simulink model "motor_kit_sim_20MHz"  (R2021b)
settings: Solver=VariableStepAuto  StartTime=0.0  StopTime=10*62.5E-6  RelTol=1e-3  EnableMultiTasking=on
PreLoadFcn:
  | setup_motor_kit_sim_20MHz;
InitFcn:
  | setup_motor_kit_sim_20MHz;
values from neighbouring files (symbols this model uses):
  DSPBASampleTime = 0.05e-6    (= 5e-08)    [setup_motor_kit_sim_20MHz.m]
  wordLength = 16    [setup_motor_kit_sim_20MHz.m]
undefined symbols (not defined in the file or in its folder): AdvDSPBChannelOutDisplay, dpoly, dspba_ChannelInVis, dspba_ChannelOutVis, dspba_internal_get_channel_ports, evalAionMaskParam, latency, primtype, value, x
libraries: DSPBAPrim x324, DSPBAModelBus x25, DSPBABase x7, dspsrcs4 x3, simulink x3, DSPBAUtilities x1
(part 2 of 5)

== system motor_kit_sim_20MHz/MotorModel/Current_scale_64_2 ==
  note: Motor phase currents 16 bits Sigma-Delta ADC (ADC interface:16 bits . Interface rtl: ip\ssg_emb_sd_adc ) : 1024 counts/A. Data type:sfix16_En10. Convert this value to range 0 to 1 (ufix16_En16). 2^16/1024 = 64; 2^15/1024 = 32. This means -32A will be 0 and 32A will be 1.
      | Schematic page 12: +/-32A current measurement. Current is sensed across 0.01 resistor. I=V/R = V/0.01 = 100*V
      | Motor phase currents Intel MAX10 ADC: 81.9 counts/A, convert this value to 16 bits, same as Sigma-Delta ADC:
      | MAX10 ADC read back value * 1024/81.9 = MAX10 ADC read back value * 12803/1024
  Current_range_int16 : Inport
  Current_sfix16_En10 : Inport  Port=2
  Add1 : DSPBAPrim/Add  primtype=add  nInputs=evalAionMaskParam(gcb,'value',1)  nOutputs=1  omode=Inherit via internal rule with word growth  otype=sfix(16)  scale=2^-15  rndmethod=Unbiased  factor=1  satmethod=Symmetric  shift_vec=[0 1 2 -1]  value=2  inPortNames=[' '; ' ';]  outPortNames=[' ']  dspbaimage=dspba_prim.svg  text=fprintf('+');  style=Optimised  visibilities=1032+2^17+2^18+2^19  genFPC=off  floatRounding=correct  advOptions=[]  version=20211007
  Const1 : DSPBAPrim/Const  primtype=const  nInputs=0  nOutputs=1  omode=Specify via dialog  otype=DataType  scale=constScaleFraction  rndmethod=Unbiased  factor=1  satmethod=Symmetric  shift_vec=[0 1 2 -1]  value=1/2  inPortNames=['+'; '+';]  outPortNames=[' ']  dspbaimage=dspba_prim.svg  text=fprintf('%s', num2str(value));  style=Optimised  visibilities=8 + 1024  floatPrecision=float32_m23  warnSaturation=on  version=20211007  SampleTime=inf
  Convert4 : DSPBAPrim/Convert  primtype=convert  nInputs=1  nOutputs=1  omode=Specify via dialog  otype=DataTypeFraction  scale=constScaleFraction  rndmethod=Biased  factor=1  satmethod=None  shift_vec=[0 1 2 -1]  value=round([0:255]/17)  inPortNames=[' '; ' ';]  outPortNames=[' '; 'c']  dspbaimage=dspba_prim_wide.svg  text=fprintf('convert');  style=Optimised  visibilities=8+64+256+2^17  clipdetect=off  floatPrecision=float32_m23  advOptions=[]  version=20211007
  Divide : DSPBAPrim/Divide  primtype=divide  nInputs=2  nOutputs=1  omode=Inherit via internal rule  otype=sfix(16)  scale=2^-15  rndmethod=Unbiased  factor=1  satmethod=Symmetric  shift_vec=[0 1 2 -1]  value=round([0:255]/17)  inPortNames=[' '; ' ';]  outPortNames=[' ']  dspbaimage=dspba_prim.svg  text=fprintf('a\n----\nb');  style=Optimised  visibilities=8+2^17+2^18  floatRounding=correct  intDivider=off  advOptions=[]  version=20211007
  GPIn : DSPBAPrim/GPIn  primtype=gpin  nInputs=evalAionMaskParam(gcb,'value',1)  nOutputs=evalAionMaskParam(gcb,'value',1)  omode=Inherit via internal rule  otype=sfix(16)  scale=2^-15  rndmethod=Unbiased  factor=1  satmethod=Symmetric  shift_vec=[0 1 2 -1]  value=1  inPortNames=[' ' ' ' ' ' ' ' ' ' ' ' ' ' ' ' ' ' ' ' ' ' ' ' ' ' ' ' ' ' ' ' ' ' ' ' ' ' ' ' ' ' ' ' ' ' ' ' ' ' ' ' ' ' ' ' ' ' ' ' ' ' ' ' ' ' ' ' ' ']'  outPortNames=[' ' ' ' ' ' ' ' ' ' ' ' ' ' ' ' ' ' ' ' ' ' ' ' ' ' ' ' ' ' ' ' ' ' ' ' ' ' ' ' ' ' ' ' ' ' ' ' ' ' ' ' ' ' ' ' ' ' ' ' ' ' ' ' ' ' ' ' ' ']'  dspbaimage=dspba_prim_channel_tall.svg  text=fprintf('GPIn');  style=Optimised  visibilities=1024  scheduleOrigin=off  version=20211214
  GPIn1 : DSPBAPrim/GPIn  primtype=gpin  nInputs=evalAionMaskParam(gcb,'value',1)  nOutputs=evalAionMaskParam(gcb,'value',1)  omode=Inherit via internal rule  otype=sfix(16)  scale=2^-15  rndmethod=Unbiased  factor=1  satmethod=Symmetric  shift_vec=[0 1 2 -1]  value=1  inPortNames=[' ' ' ' ' ' ' ' ' ' ' ' ' ' ' ' ' ' ' ' ' ' ' ' ' ' ' ' ' ' ' ' ' ' ' ' ' ' ' ' ' ' ' ' ' ' ' ' ' ' ' ' ' ' ' ' ' ' ' ' ' ' ' ' ' ' ' ' ' ']'  outPortNames=[' ' ' ' ' ' ' ' ' ' ' ' ' ' ' ' ' ' ' ' ' ' ' ' ' ' ' ' ' ' ' ' ' ' ' ' ' ' ' ' ' ' ' ' ' ' ' ' ' ' ' ' ' ' ' ' ' ' ' ' ' ' ' ' ' ' ' ' ' ']'  dspbaimage=dspba_prim_channel_tall.svg  text=fprintf('GPIn');  style=Optimised  visibilities=1024  scheduleOrigin=off  version=20211214
  GPOut : DSPBAPrim/GPOut  primtype=gpout  nInputs=evalAionMaskParam(gcb,'value',1)  nOutputs=evalAionMaskParam(gcb,'value',1)  omode=Inherit via internal rule  otype=sfix(16)  scale=2^-15  rndmethod=Unbiased  factor=1  satmethod=Symmetric  shift_vec=[0 1 2 -1]  value=1  inPortNames=[' ' ' ' ' ' ' ' ' ' ' ' ' ' ' ' ' ' ' ' ' ' ' ' ' ' ' ' ' ' ' ' ' ' ' ' ' ' ' ' ' ' ' ' ' ' ' ' ' ' ' ' ' ' ' ' ' ' ' ' ' ' ' ' ' ' ' ' ' ']'  outPortNames=[' ' ' ' ' ' ' ' ' ' ' ' ' ' ' ' ' ' ' ' ' ' ' ' ' ' ' ' ' ' ' ' ' ' ' ' ' ' ' ' ' ' ' ' ' ' ' ' ' ' ' ' ' ' ' ' ' ' ' ' ' ' ' ' ' ' ' ' ' ']'  dspbaimage=dspba_prim_channel_tall.svg  text=fprintf('GPOut');  style=Optimised  visibilities=1024  latency=13  version=20211214
  Mult : DSPBAPrim/Mult  primtype=mult  nInputs=2  nOutputs=1  omode=Inherit via internal rule  otype=sfix(16)  scale=2^-15  rndmethod=Unbiased  factor=1  satmethod=Symmetric  shift_vec=[0 1 2 -1]  value=0  inPortNames=[' '; ' ';]  outPortNames=[' ']  dspbaimage=dspba_prim.svg  text=fprintf('X');  style=Optimised  visibilities=8+2^18+2^19  floatPrecision=float32_m23  floatRounding=correct  advOptions=[]  version=20211007
  SynthesisInfo1 : DSPBAPrim/SynthesisInfo  primtype=synthinfo  nInputs=0  nOutputs=0  omode=Inherit via internal rule  otype=sfix(16)  scale=2^-15  rndmethod=Truncate  factor=1  satmethod=Symmetric  shift_vec=[0 1 2 -1]  value=99  inPortNames=[' '; ' ';]  outPortNames=[' ']  dspbaimage=dspba_prim_ctrl.jpg  text=fprintf('Style=%s', style);  style=Scheduled  visibilities=2^17+2^18+2^19+2^20  constraintPair=None  constraintRelation=>  constraintLimit=2  modelRefSign=+  modelRef=''  showSchedule=off  simulationMode=Use Global Value  resetMinimization=Conditional - On for ChannelIn/Out only  version=20220106
  "Fraction_ND_ufix16_En16 " : Outport
  wires:
  Mult/1 -> Convert4/1
  GPIn1/1 -> Add1/2
  Divide/1 -> Mult/1
  Current_range_int16/1 -> GPIn/1
  Add1/1 -> Mult/2
  Convert4/1 -> GPOut/1
  GPOut/1 -> "Fraction_ND_ufix16_En16 "/1
  GPIn/1 -> Divide/2, Add1/1
  Const1/1 -> Divide/1
  Current_sfix16_En10/1 -> GPIn1/1

== system motor_kit_sim_20MHz/MotorModel/Fraction_to_Pulse ==
  note: Subtract threshold once it is reached
  Fraction_ND_ufix16_En16 : Inport
  Add : DSPBAPrim/Add  primtype=add  nInputs=evalAionMaskParam(gcb,'value',1)  nOutputs=1  omode=Inherit via internal rule with word growth  otype=sfix(16)  scale=2^-15  rndmethod=Unbiased  factor=1  satmethod=Symmetric  shift_vec=[0 1 2 -1]  value=2  inPortNames=[' '; ' ';]  outPortNames=[' ']  dspbaimage=dspba_prim.svg  text=fprintf('+');  style=Optimised  visibilities=1032+2^17+2^18+2^19  genFPC=off  floatRounding=correct  advOptions=[]  version=20211007
  CmpGE : DSPBAPrim/CmpGE  primtype=cmpgte  nInputs=2  nOutputs=1  omode=boolean  otype=sfix(16)  scale=2^-15  rndmethod=Unbiased  factor=1  satmethod=Symmetric  shift_vec=[0 1 2 -1]  value=0  inPortNames=['a'; 'b';]  outPortNames=[' ']  dspbaimage=dspba_prim.svg  text=fprintf('a>=b');  style=Optimised  visibilities=0  advOptions=[]  version=20211007
  Const1 : DSPBAPrim/Const  primtype=const  nInputs=0  nOutputs=1  omode=Specify via dialog  otype=DataTypeFraction  scale=constScaleFraction  rndmethod=Unbiased  factor=1  satmethod=Symmetric  shift_vec=[0 1 2 -1]  value=1  inPortNames=['+'; '+';]  outPortNames=[' ']  dspbaimage=dspba_prim.svg  text=fprintf('%s', num2str(value));  style=Optimised  visibilities=8 + 1024  floatPrecision=float32_m23  warnSaturation=on  version=20211007  SampleTime=inf
  Const2 : DSPBAPrim/Const  primtype=const  nInputs=0  nOutputs=1  omode=Specify via dialog  otype=DataTypeFraction  scale=constScaleFraction  rndmethod=Unbiased  factor=1  satmethod=Symmetric  shift_vec=[0 1 2 -1]  value=0  inPortNames=['+'; '+';]  outPortNames=[' ']  dspbaimage=dspba_prim.svg  text=fprintf('%s', num2str(value));  style=Optimised  visibilities=8 + 1024  floatPrecision=float32_m23  warnSaturation=on  version=20211007  SampleTime=inf
  Const3 : DSPBAPrim/Const  primtype=const  nInputs=0  nOutputs=1  omode=Specify via dialog  otype=DataTypeFraction  scale=constScaleFraction  rndmethod=Unbiased  factor=1  satmethod=Symmetric  shift_vec=[0 1 2 -1]  value=1  inPortNames=['+'; '+';]  outPortNames=[' ']  dspbaimage=dspba_prim.svg  text=fprintf('%s', num2str(value));  style=Optimised  visibilities=8 + 1024  floatPrecision=float32_m23  warnSaturation=on  version=20211007  SampleTime=inf
  Convert4 : DSPBAPrim/Convert  primtype=convert  nInputs=1  nOutputs=1  omode=Specify via dialog  otype=sfix(18)  scale=constScaleFraction  rndmethod=Biased  factor=1  satmethod=None  shift_vec=[0 1 2 -1]  value=round([0:255]/17)  inPortNames=[' '; ' ';]  outPortNames=[' '; 'c']  dspbaimage=dspba_prim_wide.svg  text=fprintf('convert');  style=Optimised  visibilities=8+64+256+2^17  clipdetect=off  floatPrecision=float32_m23  advOptions=[]  version=20211007
  GPIn : DSPBAPrim/GPIn  primtype=gpin  nInputs=evalAionMaskParam(gcb,'value',1)  nOutputs=evalAionMaskParam(gcb,'value',1)  omode=Inherit via internal rule  otype=sfix(16)  scale=2^-15  rndmethod=Unbiased  factor=1  satmethod=Symmetric  shift_vec=[0 1 2 -1]  value=1  inPortNames=[' ' ' ' ' ' ' ' ' ' ' ' ' ' ' ' ' ' ' ' ' ' ' ' ' ' ' ' ' ' ' ' ' ' ' ' ' ' ' ' ' ' ' ' ' ' ' ' ' ' ' ' ' ' ' ' ' ' ' ' ' ' ' ' ' ' ' ' ' ']'  outPortNames=[' ' ' ' ' ' ' ' ' ' ' ' ' ' ' ' ' ' ' ' ' ' ' ' ' ' ' ' ' ' ' ' ' ' ' ' ' ' ' ' ' ' ' ' ' ' ' ' ' ' ' ' ' ' ' ' ' ' ' ' ' ' ' ' ' ' ' ' ' ']'  dspbaimage=dspba_prim_channel_tall.svg  text=fprintf('GPIn');  style=Optimised  visibilities=1024  scheduleOrigin=off  version=20211214
  GPOut : DSPBAPrim/GPOut  primtype=gpout  nInputs=evalAionMaskParam(gcb,'value',1)  nOutputs=evalAionMaskParam(gcb,'value',1)  omode=Inherit via internal rule  otype=sfix(16)  scale=2^-15  rndmethod=Unbiased  factor=1  satmethod=Symmetric  shift_vec=[0 1 2 -1]  value=1  inPortNames=[' ' ' ' ' ' ' ' ' ' ' ' ' ' ' ' ' ' ' ' ' ' ' ' ' ' ' ' ' ' ' ' ' ' ' ' ' ' ' ' ' ' ' ' ' ' ' ' ' ' ' ' ' ' ' ' ' ' ' ' ' ' ' ' ' ' ' ' ' ']'  outPortNames=[' ' ' ' ' ' ' ' ' ' ' ' ' ' ' ' ' ' ' ' ' ' ' ' ' ' ' ' ' ' ' ' ' ' ' ' ' ' ' ' ' ' ' ' ' ' ' ' ' ' ' ' ' ' ' ' ' ' ' ' ' ' ' ' ' ' ' ' ' ']'  dspbaimage=dspba_prim_channel_tall.svg  text=fprintf('GPOut');  style=Optimised  visibilities=1024  latency=0  version=20211214
  Mux : DSPBAPrim/Mux  primtype=mux  nInputs=evalAionMaskParam(gcb,'value',1)+1  nOutputs=1  omode=Inherit via internal rule  otype=sfix(16)  scale=2^-15  rndmethod=Unbiased  factor=1  satmethod=Symmetric  shift_vec=[0 1 2 -1]  value=2  inPortNames=['s'; 'd0'; 'd1'; 'd2'; 'd3'; 'd4'; 'd5'; 'd6'; 'd7'; 'd8'; 'd9';]  outPortNames=[' ']  dspbaimage=dspba_prim_tall.svg  text=fprintf('%s', primtype);  style=Optimised  visibilities=1032  version=20211007
  SampleDelay : DSPBAPrim/SampleDelay  primtype=sampdelay  nInputs=1  nOutputs=1  omode=Inherit via internal rule  otype=sfix(16)  scale=2^-15  rndmethod=Unbiased  factor=1  satmethod=Symmetric  shift_vec=[0 1 2 -1]  floatPrecision=float32_m23  value=1  inPortNames=[' '; ' ';]  outPortNames=[' ']  dspbaimage=dspba_prim.svg  text=dpoly(1, eye(1,value+1), 'z')  style=Optimised  visibilities=8 + 1024 + 2^17 + 2^18  flexible=off  slackgroup=0  augmented=0  version=20211007  advOptions=[]
  Sub : DSPBAPrim/Sub  primtype=sub  nInputs=2  nOutputs=1  omode=Inherit via internal rule with word growth  otype=sfix(17)  scale=2^-15  rndmethod=Unbiased  factor=1  satmethod=Symmetric  shift_vec=[0 1 2 -1]  value=0  inPortNames=['+'; '-';]  outPortNames=[' ']  dspbaimage=dspba_prim.svg  text=fprintf('-');  style=Optimised  visibilities=8+2^17+2^18  floatRounding=correct  advOptions=[]  version=20211007
  SynthesisInfo1 : DSPBAPrim/SynthesisInfo  primtype=synthinfo  nInputs=0  nOutputs=0  omode=Inherit via internal rule  otype=sfix(16)  scale=2^-15  rndmethod=Truncate  factor=1  satmethod=Symmetric  shift_vec=[0 1 2 -1]  value=99  inPortNames=[' '; ' ';]  outPortNames=[' ']  dspbaimage=dspba_prim_ctrl.jpg  text=fprintf('Style=%s', style);  style=Scheduled  visibilities=2^17+2^18+2^19+2^20  constraintPair=None  constraintRelation=>  constraintLimit=2  modelRefSign=+  modelRef=''  showSchedule=off  simulationMode=Use Global Value  resetMinimization=Conditional - On for ChannelIn/Out only  version=20220106
  "PulseDensity_Bool " : Outport
  wires:
  Mux/1 -> Sub/2
  CmpGE/1 -> GPOut/1, Mux/1
  GPIn/1 -> Sub/1
  Const2/1 -> Mux/2
  Const1/1 -> Mux/3
  Sub/1 -> Add/1
  Fraction_ND_ufix16_En16/1 -> GPIn/1
  GPOut/1 -> "PulseDensity_Bool "/1
  Add/1 -> Convert4/1
  Const3/1 -> CmpGE/2
  SampleDelay/1 -> Add/2, CmpGE/1
  Convert4/1 -> SampleDelay/1

== system motor_kit_sim_20MHz/MotorModel/Fraction_to_Pulse1 ==
  note: Subtract threshold once it is reached
  Fraction_ND_ufix16_En16 : Inport
  Add : DSPBAPrim/Add  primtype=add  nInputs=evalAionMaskParam(gcb,'value',1)  nOutputs=1  omode=Inherit via internal rule with word growth  otype=sfix(16)  scale=2^-15  rndmethod=Unbiased  factor=1  satmethod=Symmetric  shift_vec=[0 1 2 -1]  value=2  inPortNames=[' '; ' ';]  outPortNames=[' ']  dspbaimage=dspba_prim.svg  text=fprintf('+');  style=Optimised  visibilities=1032+2^17+2^18+2^19  genFPC=off  floatRounding=correct  advOptions=[]  version=20211007
  CmpGE : DSPBAPrim/CmpGE  primtype=cmpgte  nInputs=2  nOutputs=1  omode=boolean  otype=sfix(16)  scale=2^-15  rndmethod=Unbiased  factor=1  satmethod=Symmetric  shift_vec=[0 1 2 -1]  value=0  inPortNames=['a'; 'b';]  outPortNames=[' ']  dspbaimage=dspba_prim.svg  text=fprintf('a>=b');  style=Optimised  visibilities=0  advOptions=[]  version=20211007
  Const1 : DSPBAPrim/Const  primtype=const  nInputs=0  nOutputs=1  omode=Specify via dialog  otype=DataTypeFraction  scale=constScaleFraction  rndmethod=Unbiased  factor=1  satmethod=Symmetric  shift_vec=[0 1 2 -1]  value=1  inPortNames=['+'; '+';]  outPortNames=[' ']  dspbaimage=dspba_prim.svg  text=fprintf('%s', num2str(value));  style=Optimised  visibilities=8 + 1024  floatPrecision=float32_m23  warnSaturation=on  version=20211007  SampleTime=inf
  Const2 : DSPBAPrim/Const  primtype=const  nInputs=0  nOutputs=1  omode=Specify via dialog  otype=DataTypeFraction  scale=constScaleFraction  rndmethod=Unbiased  factor=1  satmethod=Symmetric  shift_vec=[0 1 2 -1]  value=0  inPortNames=['+'; '+';]  outPortNames=[' ']  dspbaimage=dspba_prim.svg  text=fprintf('%s', num2str(value));  style=Optimised  visibilities=8 + 1024  floatPrecision=float32_m23  warnSaturation=on  version=20211007  SampleTime=inf
  Const3 : DSPBAPrim/Const  primtype=const  nInputs=0  nOutputs=1  omode=Specify via dialog  otype=DataTypeFraction  scale=constScaleFraction  rndmethod=Unbiased  factor=1  satmethod=Symmetric  shift_vec=[0 1 2 -1]  value=1  inPortNames=['+'; '+';]  outPortNames=[' ']  dspbaimage=dspba_prim.svg  text=fprintf('%s', num2str(value));  style=Optimised  visibilities=8 + 1024  floatPrecision=float32_m23  warnSaturation=on  version=20211007  SampleTime=inf
  Convert4 : DSPBAPrim/Convert  primtype=convert  nInputs=1  nOutputs=1  omode=Specify via dialog  otype=sfix(18)  scale=constScaleFraction  rndmethod=Biased  factor=1  satmethod=None  shift_vec=[0 1 2 -1]  value=round([0:255]/17)  inPortNames=[' '; ' ';]  outPortNames=[' '; 'c']  dspbaimage=dspba_prim_wide.svg  text=fprintf('convert');  style=Optimised  visibilities=8+64+256+2^17  clipdetect=off  floatPrecision=float32_m23  advOptions=[]  version=20211007
  GPIn : DSPBAPrim/GPIn  primtype=gpin  nInputs=evalAionMaskParam(gcb,'value',1)  nOutputs=evalAionMaskParam(gcb,'value',1)  omode=Inherit via internal rule  otype=sfix(16)  scale=2^-15  rndmethod=Unbiased  factor=1  satmethod=Symmetric  shift_vec=[0 1 2 -1]  value=1  inPortNames=[' ' ' ' ' ' ' ' ' ' ' ' ' ' ' ' ' ' ' ' ' ' ' ' ' ' ' ' ' ' ' ' ' ' ' ' ' ' ' ' ' ' ' ' ' ' ' ' ' ' ' ' ' ' ' ' ' ' ' ' ' ' ' ' ' ' ' ' ' ']'  outPortNames=[' ' ' ' ' ' ' ' ' ' ' ' ' ' ' ' ' ' ' ' ' ' ' ' ' ' ' ' ' ' ' ' ' ' ' ' ' ' ' ' ' ' ' ' ' ' ' ' ' ' ' ' ' ' ' ' ' ' ' ' ' ' ' ' ' ' ' ' ' ']'  dspbaimage=dspba_prim_channel_tall.svg  text=fprintf('GPIn');  style=Optimised  visibilities=1024  scheduleOrigin=off  version=20211214
  GPOut : DSPBAPrim/GPOut  primtype=gpout  nInputs=evalAionMaskParam(gcb,'value',1)  nOutputs=evalAionMaskParam(gcb,'value',1)  omode=Inherit via internal rule  otype=sfix(16)  scale=2^-15  rndmethod=Unbiased  factor=1  satmethod=Symmetric  shift_vec=[0 1 2 -1]  value=1  inPortNames=[' ' ' ' ' ' ' ' ' ' ' ' ' ' ' ' ' ' ' ' ' ' ' ' ' ' ' ' ' ' ' ' ' ' ' ' ' ' ' ' ' ' ' ' ' ' ' ' ' ' ' ' ' ' ' ' ' ' ' ' ' ' ' ' ' ' ' ' ' ']'  outPortNames=[' ' ' ' ' ' ' ' ' ' ' ' ' ' ' ' ' ' ' ' ' ' ' ' ' ' ' ' ' ' ' ' ' ' ' ' ' ' ' ' ' ' ' ' ' ' ' ' ' ' ' ' ' ' ' ' ' ' ' ' ' ' ' ' ' ' ' ' ' ']'  dspbaimage=dspba_prim_channel_tall.svg  text=fprintf('GPOut');  style=Optimised  visibilities=1024  latency=0  version=20211214
  Mux : DSPBAPrim/Mux  primtype=mux  nInputs=evalAionMaskParam(gcb,'value',1)+1  nOutputs=1  omode=Inherit via internal rule  otype=sfix(16)  scale=2^-15  rndmethod=Unbiased  factor=1  satmethod=Symmetric  shift_vec=[0 1 2 -1]  value=2  inPortNames=['s'; 'd0'; 'd1'; 'd2'; 'd3'; 'd4'; 'd5'; 'd6'; 'd7'; 'd8'; 'd9';]  outPortNames=[' ']  dspbaimage=dspba_prim_tall.svg  text=fprintf('%s', primtype);  style=Optimised  visibilities=1032  version=20211007
  SampleDelay : DSPBAPrim/SampleDelay  primtype=sampdelay  nInputs=1  nOutputs=1  omode=Inherit via internal rule  otype=sfix(16)  scale=2^-15  rndmethod=Unbiased  factor=1  satmethod=Symmetric  shift_vec=[0 1 2 -1]  floatPrecision=float32_m23  value=1  inPortNames=[' '; ' ';]  outPortNames=[' ']  dspbaimage=dspba_prim.svg  text=dpoly(1, eye(1,value+1), 'z')  style=Optimised  visibilities=8 + 1024 + 2^17 + 2^18  flexible=off  slackgroup=0  augmented=0  version=20211007  advOptions=[]
  Sub : DSPBAPrim/Sub  primtype=sub  nInputs=2  nOutputs=1  omode=Inherit via internal rule with word growth  otype=sfix(17)  scale=2^-15  rndmethod=Unbiased  factor=1  satmethod=Symmetric  shift_vec=[0 1 2 -1]  value=0  inPortNames=['+'; '-';]  outPortNames=[' ']  dspbaimage=dspba_prim.svg  text=fprintf('-');  style=Optimised  visibilities=8+2^17+2^18  floatRounding=correct  advOptions=[]  version=20211007
  SynthesisInfo1 : DSPBAPrim/SynthesisInfo  primtype=synthinfo  nInputs=0  nOutputs=0  omode=Inherit via internal rule  otype=sfix(16)  scale=2^-15  rndmethod=Truncate  factor=1  satmethod=Symmetric  shift_vec=[0 1 2 -1]  value=99  inPortNames=[' '; ' ';]  outPortNames=[' ']  dspbaimage=dspba_prim_ctrl.jpg  text=fprintf('Style=%s', style);  style=Scheduled  visibilities=2^17+2^18+2^19+2^20  constraintPair=None  constraintRelation=>  constraintLimit=2  modelRefSign=+  modelRef=''  showSchedule=off  simulationMode=Use Global Value  resetMinimization=Conditional - On for ChannelIn/Out only  version=20220106
  "PulseDensity_Bool " : Outport
  wires:
  Mux/1 -> Sub/2
  CmpGE/1 -> GPOut/1, Mux/1
  GPIn/1 -> Sub/1
  Const2/1 -> Mux/2
  Const1/1 -> Mux/3
  Sub/1 -> Add/1
  Fraction_ND_ufix16_En16/1 -> GPIn/1
  GPOut/1 -> "PulseDensity_Bool "/1
  Add/1 -> Convert4/1
  Const3/1 -> CmpGE/2
  SampleDelay/1 -> Add/2, CmpGE/1
  Convert4/1 -> SampleDelay/1

== system motor_kit_sim_20MHz/MotorModel/Fraction_to_Pulse2 ==
  note: Subtract threshold once it is reached
  Fraction_ND_ufix16_En16 : Inport
  Add : DSPBAPrim/Add  primtype=add  nInputs=evalAionMaskParam(gcb,'value',1)  nOutputs=1  omode=Inherit via internal rule with word growth  otype=sfix(16)  scale=2^-15  rndmethod=Unbiased  factor=1  satmethod=Symmetric  shift_vec=[0 1 2 -1]  value=2  inPortNames=[' '; ' ';]  outPortNames=[' ']  dspbaimage=dspba_prim.svg  text=fprintf('+');  style=Optimised  visibilities=1032+2^17+2^18+2^19  genFPC=off  floatRounding=correct  advOptions=[]  version=20211007
  CmpGE : DSPBAPrim/CmpGE  primtype=cmpgte  nInputs=2  nOutputs=1  omode=boolean  otype=sfix(16)  scale=2^-15  rndmethod=Unbiased  factor=1  satmethod=Symmetric  shift_vec=[0 1 2 -1]  value=0  inPortNames=['a'; 'b';]  outPortNames=[' ']  dspbaimage=dspba_prim.svg  text=fprintf('a>=b');  style=Optimised  visibilities=0  advOptions=[]  version=20211007
  Const1 : DSPBAPrim/Const  primtype=const  nInputs=0  nOutputs=1  omode=Specify via dialog  otype=DataTypeFraction  scale=constScaleFraction  rndmethod=Unbiased  factor=1  satmethod=Symmetric  shift_vec=[0 1 2 -1]  value=1  inPortNames=['+'; '+';]  outPortNames=[' ']  dspbaimage=dspba_prim.svg  text=fprintf('%s', num2str(value));  style=Optimised  visibilities=8 + 1024  floatPrecision=float32_m23  warnSaturation=on  version=20211007  SampleTime=inf
  Const2 : DSPBAPrim/Const  primtype=const  nInputs=0  nOutputs=1  omode=Specify via dialog  otype=DataTypeFraction  scale=constScaleFraction  rndmethod=Unbiased  factor=1  satmethod=Symmetric  shift_vec=[0 1 2 -1]  value=0  inPortNames=['+'; '+';]  outPortNames=[' ']  dspbaimage=dspba_prim.svg  text=fprintf('%s', num2str(value));  style=Optimised  visibilities=8 + 1024  floatPrecision=float32_m23  warnSaturation=on  version=20211007  SampleTime=inf
  Const3 : DSPBAPrim/Const  primtype=const  nInputs=0  nOutputs=1  omode=Specify via dialog  otype=DataTypeFraction  scale=constScaleFraction  rndmethod=Unbiased  factor=1  satmethod=Symmetric  shift_vec=[0 1 2 -1]  value=1  inPortNames=['+'; '+';]  outPortNames=[' ']  dspbaimage=dspba_prim.svg  text=fprintf('%s', num2str(value));  style=Optimised  visibilities=8 + 1024  floatPrecision=float32_m23  warnSaturation=on  version=20211007  SampleTime=inf
  Convert4 : DSPBAPrim/Convert  primtype=convert  nInputs=1  nOutputs=1  omode=Specify via dialog  otype=sfix(18)  scale=constScaleFraction  rndmethod=Biased  factor=1  satmethod=None  shift_vec=[0 1 2 -1]  value=round([0:255]/17)  inPortNames=[' '; ' ';]  outPortNames=[' '; 'c']  dspbaimage=dspba_prim_wide.svg  text=fprintf('convert');  style=Optimised  visibilities=8+64+256+2^17  clipdetect=off  floatPrecision=float32_m23  advOptions=[]  version=20211007
  GPIn : DSPBAPrim/GPIn  primtype=gpin  nInputs=evalAionMaskParam(gcb,'value',1)  nOutputs=evalAionMaskParam(gcb,'value',1)  omode=Inherit via internal rule  otype=sfix(16)  scale=2^-15  rndmethod=Unbiased  factor=1  satmethod=Symmetric  shift_vec=[0 1 2 -1]  value=1  inPortNames=[' ' ' ' ' ' ' ' ' ' ' ' ' ' ' ' ' ' ' ' ' ' ' ' ' ' ' ' ' ' ' ' ' ' ' ' ' ' ' ' ' ' ' ' ' ' ' ' ' ' ' ' ' ' ' ' ' ' ' ' ' ' ' ' ' ' ' ' ' ']'  outPortNames=[' ' ' ' ' ' ' ' ' ' ' ' ' ' ' ' ' ' ' ' ' ' ' ' ' ' ' ' ' ' ' ' ' ' ' ' ' ' ' ' ' ' ' ' ' ' ' ' ' ' ' ' ' ' ' ' ' ' ' ' ' ' ' ' ' ' ' ' ' ']'  dspbaimage=dspba_prim_channel_tall.svg  text=fprintf('GPIn');  style=Optimised  visibilities=1024  scheduleOrigin=off  version=20211214
  GPOut : DSPBAPrim/GPOut  primtype=gpout  nInputs=evalAionMaskParam(gcb,'value',1)  nOutputs=evalAionMaskParam(gcb,'value',1)  omode=Inherit via internal rule  otype=sfix(16)  scale=2^-15  rndmethod=Unbiased  factor=1  satmethod=Symmetric  shift_vec=[0 1 2 -1]  value=1  inPortNames=[' ' ' ' ' ' ' ' ' ' ' ' ' ' ' ' ' ' ' ' ' ' ' ' ' ' ' ' ' ' ' ' ' ' ' ' ' ' ' ' ' ' ' ' ' ' ' ' ' ' ' ' ' ' ' ' ' ' ' ' ' ' ' ' ' ' ' ' ' ']'  outPortNames=[' ' ' ' ' ' ' ' ' ' ' ' ' ' ' ' ' ' ' ' ' ' ' ' ' ' ' ' ' ' ' ' ' ' ' ' ' ' ' ' ' ' ' ' ' ' ' ' ' ' ' ' ' ' ' ' ' ' ' ' ' ' ' ' ' ' ' ' ' ']'  dspbaimage=dspba_prim_channel_tall.svg  text=fprintf('GPOut');  style=Optimised  visibilities=1024  latency=0  version=20211214
  Mux : DSPBAPrim/Mux  primtype=mux  nInputs=evalAionMaskParam(gcb,'value',1)+1  nOutputs=1  omode=Inherit via internal rule  otype=sfix(16)  scale=2^-15  rndmethod=Unbiased  factor=1  satmethod=Symmetric  shift_vec=[0 1 2 -1]  value=2  inPortNames=['s'; 'd0'; 'd1'; 'd2'; 'd3'; 'd4'; 'd5'; 'd6'; 'd7'; 'd8'; 'd9';]  outPortNames=[' ']  dspbaimage=dspba_prim_tall.svg  text=fprintf('%s', primtype);  style=Optimised  visibilities=1032  version=20211007
  SampleDelay : DSPBAPrim/SampleDelay  primtype=sampdelay  nInputs=1  nOutputs=1  omode=Inherit via internal rule  otype=sfix(16)  scale=2^-15  rndmethod=Unbiased  factor=1  satmethod=Symmetric  shift_vec=[0 1 2 -1]  floatPrecision=float32_m23  value=1  inPortNames=[' '; ' ';]  outPortNames=[' ']  dspbaimage=dspba_prim.svg  text=dpoly(1, eye(1,value+1), 'z')  style=Optimised  visibilities=8 + 1024 + 2^17 + 2^18  flexible=off  slackgroup=0  augmented=0  version=20211007  advOptions=[]
  Sub : DSPBAPrim/Sub  primtype=sub  nInputs=2  nOutputs=1  omode=Inherit via internal rule with word growth  otype=sfix(17)  scale=2^-15  rndmethod=Unbiased  factor=1  satmethod=Symmetric  shift_vec=[0 1 2 -1]  value=0  inPortNames=['+'; '-';]  outPortNames=[' ']  dspbaimage=dspba_prim.svg  text=fprintf('-');  style=Optimised  visibilities=8+2^17+2^18  floatRounding=correct  advOptions=[]  version=20211007
  SynthesisInfo1 : DSPBAPrim/SynthesisInfo  primtype=synthinfo  nInputs=0  nOutputs=0  omode=Inherit via internal rule  otype=sfix(16)  scale=2^-15  rndmethod=Truncate  factor=1  satmethod=Symmetric  shift_vec=[0 1 2 -1]  value=99  inPortNames=[' '; ' ';]  outPortNames=[' ']  dspbaimage=dspba_prim_ctrl.jpg  text=fprintf('Style=%s', style);  style=Scheduled  visibilities=2^17+2^18+2^19+2^20  constraintPair=None  constraintRelation=>  constraintLimit=2  modelRefSign=+  modelRef=''  showSchedule=off  simulationMode=Use Global Value  resetMinimization=Conditional - On for ChannelIn/Out only  version=20220106
  "PulseDensity_Bool " : Outport
  wires:
  Mux/1 -> Sub/2
  CmpGE/1 -> GPOut/1, Mux/1
  GPIn/1 -> Sub/1
  Const2/1 -> Mux/2
  Const1/1 -> Mux/3
  Sub/1 -> Add/1
  Fraction_ND_ufix16_En16/1 -> GPIn/1
  GPOut/1 -> "PulseDensity_Bool "/1
  Add/1 -> Convert4/1
  Const3/1 -> CmpGE/2
  SampleDelay/1 -> Add/2, CmpGE/1
  Convert4/1 -> SampleDelay/1

== system motor_kit_sim_20MHz/MotorModel/Fraction_to_Pulse3 ==
  note: Subtract threshold once it is reached
  Fraction_ND_ufix16_En16 : Inport
  Add : DSPBAPrim/Add  primtype=add  nInputs=evalAionMaskParam(gcb,'value',1)  nOutputs=1  omode=Inherit via internal rule with word growth  otype=sfix(16)  scale=2^-15  rndmethod=Unbiased  factor=1  satmethod=Symmetric  shift_vec=[0 1 2 -1]  value=2  inPortNames=[' '; ' ';]  outPortNames=[' ']  dspbaimage=dspba_prim.svg  text=fprintf('+');  style=Optimised  visibilities=1032+2^17+2^18+2^19  genFPC=off  floatRounding=correct  advOptions=[]  version=20211007
  CmpGE : DSPBAPrim/CmpGE  primtype=cmpgte  nInputs=2  nOutputs=1  omode=boolean  otype=sfix(16)  scale=2^-15  rndmethod=Unbiased  factor=1  satmethod=Symmetric  shift_vec=[0 1 2 -1]  value=0  inPortNames=['a'; 'b';]  outPortNames=[' ']  dspbaimage=dspba_prim.svg  text=fprintf('a>=b');  style=Optimised  visibilities=0  advOptions=[]  version=20211007
  Const1 : DSPBAPrim/Const  primtype=const  nInputs=0  nOutputs=1  omode=Specify via dialog  otype=DataTypeFraction  scale=constScaleFraction  rndmethod=Unbiased  factor=1  satmethod=Symmetric  shift_vec=[0 1 2 -1]  value=1  inPortNames=['+'; '+';]  outPortNames=[' ']  dspbaimage=dspba_prim.svg  text=fprintf('%s', num2str(value));  style=Optimised  visibilities=8 + 1024  floatPrecision=float32_m23  warnSaturation=on  version=20211007  SampleTime=inf
  Const2 : DSPBAPrim/Const  primtype=const  nInputs=0  nOutputs=1  omode=Specify via dialog  otype=DataTypeFraction  scale=constScaleFraction  rndmethod=Unbiased  factor=1  satmethod=Symmetric  shift_vec=[0 1 2 -1]  value=0  inPortNames=['+'; '+';]  outPortNames=[' ']  dspbaimage=dspba_prim.svg  text=fprintf('%s', num2str(value));  style=Optimised  visibilities=8 + 1024  floatPrecision=float32_m23  warnSaturation=on  version=20211007  SampleTime=inf
  Const3 : DSPBAPrim/Const  primtype=const  nInputs=0  nOutputs=1  omode=Specify via dialog  otype=DataTypeFraction  scale=constScaleFraction  rndmethod=Unbiased  factor=1  satmethod=Symmetric  shift_vec=[0 1 2 -1]  value=1  inPortNames=['+'; '+';]  outPortNames=[' ']  dspbaimage=dspba_prim.svg  text=fprintf('%s', num2str(value));  style=Optimised  visibilities=8 + 1024  floatPrecision=float32_m23  warnSaturation=on  version=20211007  SampleTime=inf
  Convert4 : DSPBAPrim/Convert  primtype=convert  nInputs=1  nOutputs=1  omode=Specify via dialog  otype=sfix(18)  scale=constScaleFraction  rndmethod=Biased  factor=1  satmethod=None  shift_vec=[0 1 2 -1]  value=round([0:255]/17)  inPortNames=[' '; ' ';]  outPortNames=[' '; 'c']  dspbaimage=dspba_prim_wide.svg  text=fprintf('convert');  style=Optimised  visibilities=8+64+256+2^17  clipdetect=off  floatPrecision=float32_m23  advOptions=[]  version=20211007
  GPIn : DSPBAPrim/GPIn  primtype=gpin  nInputs=evalAionMaskParam(gcb,'value',1)  nOutputs=evalAionMaskParam(gcb,'value',1)  omode=Inherit via internal rule  otype=sfix(16)  scale=2^-15  rndmethod=Unbiased  factor=1  satmethod=Symmetric  shift_vec=[0 1 2 -1]  value=1  inPortNames=[' ' ' ' ' ' ' ' ' ' ' ' ' ' ' ' ' ' ' ' ' ' ' ' ' ' ' ' ' ' ' ' ' ' ' ' ' ' ' ' ' ' ' ' ' ' ' ' ' ' ' ' ' ' ' ' ' ' ' ' ' ' ' ' ' ' ' ' ' ']'  outPortNames=[' ' ' ' ' ' ' ' ' ' ' ' ' ' ' ' ' ' ' ' ' ' ' ' ' ' ' ' ' ' ' ' ' ' ' ' ' ' ' ' ' ' ' ' ' ' ' ' ' ' ' ' ' ' ' ' ' ' ' ' ' ' ' ' ' ' ' ' ' ']'  dspbaimage=dspba_prim_channel_tall.svg  text=fprintf('GPIn');  style=Optimised  visibilities=1024  scheduleOrigin=off  version=20211214
  GPOut : DSPBAPrim/GPOut  primtype=gpout  nInputs=evalAionMaskParam(gcb,'value',1)  nOutputs=evalAionMaskParam(gcb,'value',1)  omode=Inherit via internal rule  otype=sfix(16)  scale=2^-15  rndmethod=Unbiased  factor=1  satmethod=Symmetric  shift_vec=[0 1 2 -1]  value=1  inPortNames=[' ' ' ' ' ' ' ' ' ' ' ' ' ' ' ' ' ' ' ' ' ' ' ' ' ' ' ' ' ' ' ' ' ' ' ' ' ' ' ' ' ' ' ' ' ' ' ' ' ' ' ' ' ' ' ' ' ' ' ' ' ' ' ' ' ' ' ' ' ']'  outPortNames=[' ' ' ' ' ' ' ' ' ' ' ' ' ' ' ' ' ' ' ' ' ' ' ' ' ' ' ' ' ' ' ' ' ' ' ' ' ' ' ' ' ' ' ' ' ' ' ' ' ' ' ' ' ' ' ' ' ' ' ' ' ' ' ' ' ' ' ' ' ']'  dspbaimage=dspba_prim_channel_tall.svg  text=fprintf('GPOut');  style=Optimised  visibilities=1024  latency=0  version=20211214
  Mux : DSPBAPrim/Mux  primtype=mux  nInputs=evalAionMaskParam(gcb,'value',1)+1  nOutputs=1  omode=Inherit via internal rule  otype=sfix(16)  scale=2^-15  rndmethod=Unbiased  factor=1  satmethod=Symmetric  shift_vec=[0 1 2 -1]  value=2  inPortNames=['s'; 'd0'; 'd1'; 'd2'; 'd3'; 'd4'; 'd5'; 'd6'; 'd7'; 'd8'; 'd9';]  outPortNames=[' ']  dspbaimage=dspba_prim_tall.svg  text=fprintf('%s', primtype);  style=Optimised  visibilities=1032  version=20211007
  SampleDelay : DSPBAPrim/SampleDelay  primtype=sampdelay  nInputs=1  nOutputs=1  omode=Inherit via internal rule  otype=sfix(16)  scale=2^-15  rndmethod=Unbiased  factor=1  satmethod=Symmetric  shift_vec=[0 1 2 -1]  floatPrecision=float32_m23  value=1  inPortNames=[' '; ' ';]  outPortNames=[' ']  dspbaimage=dspba_prim.svg  text=dpoly(1, eye(1,value+1), 'z')  style=Optimised  visibilities=8 + 1024 + 2^17 + 2^18  flexible=off  slackgroup=0  augmented=0  version=20211007  advOptions=[]
  Sub : DSPBAPrim/Sub  primtype=sub  nInputs=2  nOutputs=1  omode=Inherit via internal rule with word growth  otype=sfix(17)  scale=2^-15  rndmethod=Unbiased  factor=1  satmethod=Symmetric  shift_vec=[0 1 2 -1]  value=0  inPortNames=['+'; '-';]  outPortNames=[' ']  dspbaimage=dspba_prim.svg  text=fprintf('-');  style=Optimised  visibilities=8+2^17+2^18  floatRounding=correct  advOptions=[]  version=20211007
  SynthesisInfo1 : DSPBAPrim/SynthesisInfo  primtype=synthinfo  nInputs=0  nOutputs=0  omode=Inherit via internal rule  otype=sfix(16)  scale=2^-15  rndmethod=Truncate  factor=1  satmethod=Symmetric  shift_vec=[0 1 2 -1]  value=99  inPortNames=[' '; ' ';]  outPortNames=[' ']  dspbaimage=dspba_prim_ctrl.jpg  text=fprintf('Style=%s', style);  style=Scheduled  visibilities=2^17+2^18+2^19+2^20  constraintPair=None  constraintRelation=>  constraintLimit=2  modelRefSign=+  modelRef=''  showSchedule=off  simulationMode=Use Global Value  resetMinimization=Conditional - On for ChannelIn/Out only  version=20220106
  "PulseDensity_Bool " : Outport
  wires:
  Mux/1 -> Sub/2
  CmpGE/1 -> GPOut/1, Mux/1
  GPIn/1 -> Sub/1
  Const2/1 -> Mux/2
  Const1/1 -> Mux/3
  Sub/1 -> Add/1
  Fraction_ND_ufix16_En16/1 -> GPIn/1
  GPOut/1 -> "PulseDensity_Bool "/1
  Add/1 -> Convert4/1
  Const3/1 -> CmpGE/2
  SampleDelay/1 -> Add/2, CmpGE/1
  Convert4/1 -> SampleDelay/1

== system motor_kit_sim_20MHz/MotorModel/Fraction_to_Pulse4 ==
  note: Subtract threshold once it is reached
  Fraction_ND_ufix16_En16 : Inport
  Add : DSPBAPrim/Add  primtype=add  nInputs=evalAionMaskParam(gcb,'value',1)  nOutputs=1  omode=Inherit via internal rule with word growth  otype=sfix(16)  scale=2^-15  rndmethod=Unbiased  factor=1  satmethod=Symmetric  shift_vec=[0 1 2 -1]  value=2  inPortNames=[' '; ' ';]  outPortNames=[' ']  dspbaimage=dspba_prim.svg  text=fprintf('+');  style=Optimised  visibilities=1032+2^17+2^18+2^19  genFPC=off  floatRounding=correct  advOptions=[]  version=20211007
  CmpGE : DSPBAPrim/CmpGE  primtype=cmpgte  nInputs=2  nOutputs=1  omode=boolean  otype=sfix(16)  scale=2^-15  rndmethod=Unbiased  factor=1  satmethod=Symmetric  shift_vec=[0 1 2 -1]  value=0  inPortNames=['a'; 'b';]  outPortNames=[' ']  dspbaimage=dspba_prim.svg  text=fprintf('a>=b');  style=Optimised  visibilities=0  advOptions=[]  version=20211007
  Const1 : DSPBAPrim/Const  primtype=const  nInputs=0  nOutputs=1  omode=Specify via dialog  otype=DataTypeFraction  scale=constScaleFraction  rndmethod=Unbiased  factor=1  satmethod=Symmetric  shift_vec=[0 1 2 -1]  value=1  inPortNames=['+'; '+';]  outPortNames=[' ']  dspbaimage=dspba_prim.svg  text=fprintf('%s', num2str(value));  style=Optimised  visibilities=8 + 1024  floatPrecision=float32_m23  warnSaturation=on  version=20211007  SampleTime=inf
  Const2 : DSPBAPrim/Const  primtype=const  nInputs=0  nOutputs=1  omode=Specify via dialog  otype=DataTypeFraction  scale=constScaleFraction  rndmethod=Unbiased  factor=1  satmethod=Symmetric  shift_vec=[0 1 2 -1]  value=0  inPortNames=['+'; '+';]  outPortNames=[' ']  dspbaimage=dspba_prim.svg  text=fprintf('%s', num2str(value));  style=Optimised  visibilities=8 + 1024  floatPrecision=float32_m23  warnSaturation=on  version=20211007  SampleTime=inf
  Const3 : DSPBAPrim/Const  primtype=const  nInputs=0  nOutputs=1  omode=Specify via dialog  otype=DataTypeFraction  scale=constScaleFraction  rndmethod=Unbiased  factor=1  satmethod=Symmetric  shift_vec=[0 1 2 -1]  value=1  inPortNames=['+'; '+';]  outPortNames=[' ']  dspbaimage=dspba_prim.svg  text=fprintf('%s', num2str(value));  style=Optimised  visibilities=8 + 1024  floatPrecision=float32_m23  warnSaturation=on  version=20211007  SampleTime=inf
  Convert4 : DSPBAPrim/Convert  primtype=convert  nInputs=1  nOutputs=1  omode=Specify via dialog  otype=sfix(18)  scale=constScaleFraction  rndmethod=Biased  factor=1  satmethod=None  shift_vec=[0 1 2 -1]  value=round([0:255]/17)  inPortNames=[' '; ' ';]  outPortNames=[' '; 'c']  dspbaimage=dspba_prim_wide.svg  text=fprintf('convert');  style=Optimised  visibilities=8+64+256+2^17  clipdetect=off  floatPrecision=float32_m23  advOptions=[]  version=20211007
  GPIn : DSPBAPrim/GPIn  primtype=gpin  nInputs=evalAionMaskParam(gcb,'value',1)  nOutputs=evalAionMaskParam(gcb,'value',1)  omode=Inherit via internal rule  otype=sfix(16)  scale=2^-15  rndmethod=Unbiased  factor=1  satmethod=Symmetric  shift_vec=[0 1 2 -1]  value=1  inPortNames=[' ' ' ' ' ' ' ' ' ' ' ' ' ' ' ' ' ' ' ' ' ' ' ' ' ' ' ' ' ' ' ' ' ' ' ' ' ' ' ' ' ' ' ' ' ' ' ' ' ' ' ' ' ' ' ' ' ' ' ' ' ' ' ' ' ' ' ' ' ']'  outPortNames=[' ' ' ' ' ' ' ' ' ' ' ' ' ' ' ' ' ' ' ' ' ' ' ' ' ' ' ' ' ' ' ' ' ' ' ' ' ' ' ' ' ' ' ' ' ' ' ' ' ' ' ' ' ' ' ' ' ' ' ' ' ' ' ' ' ' ' ' ' ']'  dspbaimage=dspba_prim_channel_tall.svg  text=fprintf('GPIn');  style=Optimised  visibilities=1024  scheduleOrigin=off  version=20211214
  GPOut : DSPBAPrim/GPOut  primtype=gpout  nInputs=evalAionMaskParam(gcb,'value',1)  nOutputs=evalAionMaskParam(gcb,'value',1)  omode=Inherit via internal rule  otype=sfix(16)  scale=2^-15  rndmethod=Unbiased  factor=1  satmethod=Symmetric  shift_vec=[0 1 2 -1]  value=1  inPortNames=[' ' ' ' ' ' ' ' ' ' ' ' ' ' ' ' ' ' ' ' ' ' ' ' ' ' ' ' ' ' ' ' ' ' ' ' ' ' ' ' ' ' ' ' ' ' ' ' ' ' ' ' ' ' ' ' ' ' ' ' ' ' ' ' ' ' ' ' ' ']'  outPortNames=[' ' ' ' ' ' ' ' ' ' ' ' ' ' ' ' ' ' ' ' ' ' ' ' ' ' ' ' ' ' ' ' ' ' ' ' ' ' ' ' ' ' ' ' ' ' ' ' ' ' ' ' ' ' ' ' ' ' ' ' ' ' ' ' ' ' ' ' ' ']'  dspbaimage=dspba_prim_channel_tall.svg  text=fprintf('GPOut');  style=Optimised  visibilities=1024  latency=0  version=20211214
  Mux : DSPBAPrim/Mux  primtype=mux  nInputs=evalAionMaskParam(gcb,'value',1)+1  nOutputs=1  omode=Inherit via internal rule  otype=sfix(16)  scale=2^-15  rndmethod=Unbiased  factor=1  satmethod=Symmetric  shift_vec=[0 1 2 -1]  value=2  inPortNames=['s'; 'd0'; 'd1'; 'd2'; 'd3'; 'd4'; 'd5'; 'd6'; 'd7'; 'd8'; 'd9';]  outPortNames=[' ']  dspbaimage=dspba_prim_tall.svg  text=fprintf('%s', primtype);  style=Optimised  visibilities=1032  version=20211007
  SampleDelay : DSPBAPrim/SampleDelay  primtype=sampdelay  nInputs=1  nOutputs=1  omode=Inherit via internal rule  otype=sfix(16)  scale=2^-15  rndmethod=Unbiased  factor=1  satmethod=Symmetric  shift_vec=[0 1 2 -1]  floatPrecision=float32_m23  value=1  inPortNames=[' '; ' ';]  outPortNames=[' ']  dspbaimage=dspba_prim.svg  text=dpoly(1, eye(1,value+1), 'z')  style=Optimised  visibilities=8 + 1024 + 2^17 + 2^18  flexible=off  slackgroup=0  augmented=0  version=20211007  advOptions=[]
  Sub : DSPBAPrim/Sub  primtype=sub  nInputs=2  nOutputs=1  omode=Inherit via internal rule with word growth  otype=sfix(17)  scale=2^-15  rndmethod=Unbiased  factor=1  satmethod=Symmetric  shift_vec=[0 1 2 -1]  value=0  inPortNames=['+'; '-';]  outPortNames=[' ']  dspbaimage=dspba_prim.svg  text=fprintf('-');  style=Optimised  visibilities=8+2^17+2^18  floatRounding=correct  advOptions=[]  version=20211007
  SynthesisInfo1 : DSPBAPrim/SynthesisInfo  primtype=synthinfo  nInputs=0  nOutputs=0  omode=Inherit via internal rule  otype=sfix(16)  scale=2^-15  rndmethod=Truncate  factor=1  satmethod=Symmetric  shift_vec=[0 1 2 -1]  value=99  inPortNames=[' '; ' ';]  outPortNames=[' ']  dspbaimage=dspba_prim_ctrl.jpg  text=fprintf('Style=%s', style);  style=Scheduled  visibilities=2^17+2^18+2^19+2^20  constraintPair=None  constraintRelation=>  constraintLimit=2  modelRefSign=+  modelRef=''  showSchedule=off  simulationMode=Use Global Value  resetMinimization=Conditional - On for ChannelIn/Out only  version=20220106
  "PulseDensity_Bool " : Outport
  wires:
  Mux/1 -> Sub/2
  CmpGE/1 -> GPOut/1, Mux/1
  GPIn/1 -> Sub/1
  Const2/1 -> Mux/2
  Const1/1 -> Mux/3
  Sub/1 -> Add/1
  Fraction_ND_ufix16_En16/1 -> GPIn/1
  GPOut/1 -> "PulseDensity_Bool "/1
  Add/1 -> Convert4/1
  Const3/1 -> CmpGE/2
  SampleDelay/1 -> Add/2, CmpGE/1
  Convert4/1 -> SampleDelay/1

== system motor_kit_sim_20MHz/MotorModel/Fraction_to_Pulse5 ==
  note: Subtract threshold once it is reached
  Fraction_ND_ufix16_En16 : Inport
  Add : DSPBAPrim/Add  primtype=add  nInputs=evalAionMaskParam(gcb,'value',1)  nOutputs=1  omode=Inherit via internal rule with word growth  otype=sfix(16)  scale=2^-15  rndmethod=Unbiased  factor=1  satmethod=Symmetric  shift_vec=[0 1 2 -1]  value=2  inPortNames=[' '; ' ';]  outPortNames=[' ']  dspbaimage=dspba_prim.svg  text=fprintf('+');  style=Optimised  visibilities=1032+2^17+2^18+2^19  genFPC=off  floatRounding=correct  advOptions=[]  version=20211007
  CmpGE : DSPBAPrim/CmpGE  primtype=cmpgte  nInputs=2  nOutputs=1  omode=boolean  otype=sfix(16)  scale=2^-15  rndmethod=Unbiased  factor=1  satmethod=Symmetric  shift_vec=[0 1 2 -1]  value=0  inPortNames=['a'; 'b';]  outPortNames=[' ']  dspbaimage=dspba_prim.svg  text=fprintf('a>=b');  style=Optimised  visibilities=0  advOptions=[]  version=20211007
  Const1 : DSPBAPrim/Const  primtype=const  nInputs=0  nOutputs=1  omode=Specify via dialog  otype=DataTypeFraction  scale=constScaleFraction  rndmethod=Unbiased  factor=1  satmethod=Symmetric  shift_vec=[0 1 2 -1]  value=1  inPortNames=['+'; '+';]  outPortNames=[' ']  dspbaimage=dspba_prim.svg  text=fprintf('%s', num2str(value));  style=Optimised  visibilities=8 + 1024  floatPrecision=float32_m23  warnSaturation=on  version=20211007  SampleTime=inf
  Const2 : DSPBAPrim/Const  primtype=const  nInputs=0  nOutputs=1  omode=Specify via dialog  otype=DataTypeFraction  scale=constScaleFraction  rndmethod=Unbiased  factor=1  satmethod=Symmetric  shift_vec=[0 1 2 -1]  value=0  inPortNames=['+'; '+';]  outPortNames=[' ']  dspbaimage=dspba_prim.svg  text=fprintf('%s', num2str(value));  style=Optimised  visibilities=8 + 1024  floatPrecision=float32_m23  warnSaturation=on  version=20211007  SampleTime=inf
  Const3 : DSPBAPrim/Const  primtype=const  nInputs=0  nOutputs=1  omode=Specify via dialog  otype=DataTypeFraction  scale=constScaleFraction  rndmethod=Unbiased  factor=1  satmethod=Symmetric  shift_vec=[0 1 2 -1]  value=1  inPortNames=['+'; '+';]  outPortNames=[' ']  dspbaimage=dspba_prim.svg  text=fprintf('%s', num2str(value));  style=Optimised  visibilities=8 + 1024  floatPrecision=float32_m23  warnSaturation=on  version=20211007  SampleTime=inf
  Convert4 : DSPBAPrim/Convert  primtype=convert  nInputs=1  nOutputs=1  omode=Specify via dialog  otype=sfix(18)  scale=constScaleFraction  rndmethod=Biased  factor=1  satmethod=None  shift_vec=[0 1 2 -1]  value=round([0:255]/17)  inPortNames=[' '; ' ';]  outPortNames=[' '; 'c']  dspbaimage=dspba_prim_wide.svg  text=fprintf('convert');  style=Optimised  visibilities=8+64+256+2^17  clipdetect=off  floatPrecision=float32_m23  advOptions=[]  version=20211007
  GPIn : DSPBAPrim/GPIn  primtype=gpin  nInputs=evalAionMaskParam(gcb,'value',1)  nOutputs=evalAionMaskParam(gcb,'value',1)  omode=Inherit via internal rule  otype=sfix(16)  scale=2^-15  rndmethod=Unbiased  factor=1  satmethod=Symmetric  shift_vec=[0 1 2 -1]  value=1  inPortNames=[' ' ' ' ' ' ' ' ' ' ' ' ' ' ' ' ' ' ' ' ' ' ' ' ' ' ' ' ' ' ' ' ' ' ' ' ' ' ' ' ' ' ' ' ' ' ' ' ' ' ' ' ' ' ' ' ' ' ' ' ' ' ' ' ' ' ' ' ' ']'  outPortNames=[' ' ' ' ' ' ' ' ' ' ' ' ' ' ' ' ' ' ' ' ' ' ' ' ' ' ' ' ' ' ' ' ' ' ' ' ' ' ' ' ' ' ' ' ' ' ' ' ' ' ' ' ' ' ' ' ' ' ' ' ' ' ' ' ' ' ' ' ' ']'  dspbaimage=dspba_prim_channel_tall.svg  text=fprintf('GPIn');  style=Optimised  visibilities=1024  scheduleOrigin=off  version=20211214
  GPOut : DSPBAPrim/GPOut  primtype=gpout  nInputs=evalAionMaskParam(gcb,'value',1)  nOutputs=evalAionMaskParam(gcb,'value',1)  omode=Inherit via internal rule  otype=sfix(16)  scale=2^-15  rndmethod=Unbiased  factor=1  satmethod=Symmetric  shift_vec=[0 1 2 -1]  value=1  inPortNames=[' ' ' ' ' ' ' ' ' ' ' ' ' ' ' ' ' ' ' ' ' ' ' ' ' ' ' ' ' ' ' ' ' ' ' ' ' ' ' ' ' ' ' ' ' ' ' ' ' ' ' ' ' ' ' ' ' ' ' ' ' ' ' ' ' ' ' ' ' ']'  outPortNames=[' ' ' ' ' ' ' ' ' ' ' ' ' ' ' ' ' ' ' ' ' ' ' ' ' ' ' ' ' ' ' ' ' ' ' ' ' ' ' ' ' ' ' ' ' ' ' ' ' ' ' ' ' ' ' ' ' ' ' ' ' ' ' ' ' ' ' ' ' ']'  dspbaimage=dspba_prim_channel_tall.svg  text=fprintf('GPOut');  style=Optimised  visibilities=1024  latency=0  version=20211214
  Mux : DSPBAPrim/Mux  primtype=mux  nInputs=evalAionMaskParam(gcb,'value',1)+1  nOutputs=1  omode=Inherit via internal rule  otype=sfix(16)  scale=2^-15  rndmethod=Unbiased  factor=1  satmethod=Symmetric  shift_vec=[0 1 2 -1]  value=2  inPortNames=['s'; 'd0'; 'd1'; 'd2'; 'd3'; 'd4'; 'd5'; 'd6'; 'd7'; 'd8'; 'd9';]  outPortNames=[' ']  dspbaimage=dspba_prim_tall.svg  text=fprintf('%s', primtype);  style=Optimised  visibilities=1032  version=20211007
  SampleDelay : DSPBAPrim/SampleDelay  primtype=sampdelay  nInputs=1  nOutputs=1  omode=Inherit via internal rule  otype=sfix(16)  scale=2^-15  rndmethod=Unbiased  factor=1  satmethod=Symmetric  shift_vec=[0 1 2 -1]  floatPrecision=float32_m23  value=1  inPortNames=[' '; ' ';]  outPortNames=[' ']  dspbaimage=dspba_prim.svg  text=dpoly(1, eye(1,value+1), 'z')  style=Optimised  visibilities=8 + 1024 + 2^17 + 2^18  flexible=off  slackgroup=0  augmented=0  version=20211007  advOptions=[]
  Sub : DSPBAPrim/Sub  primtype=sub  nInputs=2  nOutputs=1  omode=Inherit via internal rule with word growth  otype=sfix(17)  scale=2^-15  rndmethod=Unbiased  factor=1  satmethod=Symmetric  shift_vec=[0 1 2 -1]  value=0  inPortNames=['+'; '-';]  outPortNames=[' ']  dspbaimage=dspba_prim.svg  text=fprintf('-');  style=Optimised  visibilities=8+2^17+2^18  floatRounding=correct  advOptions=[]  version=20211007
  SynthesisInfo1 : DSPBAPrim/SynthesisInfo  primtype=synthinfo  nInputs=0  nOutputs=0  omode=Inherit via internal rule  otype=sfix(16)  scale=2^-15  rndmethod=Truncate  factor=1  satmethod=Symmetric  shift_vec=[0 1 2 -1]  value=99  inPortNames=[' '; ' ';]  outPortNames=[' ']  dspbaimage=dspba_prim_ctrl.jpg  text=fprintf('Style=%s', style);  style=Scheduled  visibilities=2^17+2^18+2^19+2^20  constraintPair=None  constraintRelation=>  constraintLimit=2  modelRefSign=+  modelRef=''  showSchedule=off  simulationMode=Use Global Value  resetMinimization=Conditional - On for ChannelIn/Out only  version=20220106
  "PulseDensity_Bool " : Outport
  wires:
  Mux/1 -> Sub/2
  CmpGE/1 -> GPOut/1, Mux/1
  GPIn/1 -> Sub/1
  Const2/1 -> Mux/2
  Const1/1 -> Mux/3
  Sub/1 -> Add/1
  Fraction_ND_ufix16_En16/1 -> GPIn/1
  GPOut/1 -> "PulseDensity_Bool "/1
  Add/1 -> Convert4/1
  Const3/1 -> CmpGE/2
  SampleDelay/1 -> Add/2, CmpGE/1
  Convert4/1 -> SampleDelay/1
